simulink model "main"  (R2022b)
settings: Solver=FixedStepDiscrete  StartTime=0.0  StopTime=30  FixedStep=0.005  RelTol=1e-3
libraries: lib_button x1, simulink x1
settings Model: ExtModeTrigDuration=2  Creator=F64236C  LastModifiedBy=F64236C
settings OptimizationCC: EnhancedBackFolding=on  PassReuseOutputArgsAs=Individual arguments  ZeroExternalMemoryAtStartup=off  ZeroInternalMemoryAtStartup=off  MaxStackSize=64  OptimizeBlockOrder=speed  DifferentSizesBufferReuse=on  OptimizationCustomize=off  EfficientTunableParamExpr=on
settings DebuggingCC: ParameterTunabilityLossMsg=error
settings HardwareCC: ProdBitPerInt=16  ProdBitPerPointer=16  ProdBitPerSizeT=16  ProdBitPerPtrDiffT=16  ProdLargestAtomicFloat=None  ProdWordSize=8  ProdHWDeviceType=Atmel->AVR
settings SFSimCC: MATLABDynamicMemAlloc=off
settings RTWCC: Description=Embedded Coder  SystemTargetFile=ert.tlc  HardwareBoard=Arduino Uno  TLCOptions=-aInlineSetEventsForThisBaseRateFcn=TLC_FALSE -aSuppressMultiTaskScheduler=TLC_FALSE -aRateBasedStepFcn=1  TemplateMakefile=ert_default_tmf  Toolchain=Arduino AVR  BuildConfiguration=Faster Runs
settings CodeAppCC: ForceParamTrailComments=on  IgnoreCustomStorageClasses=off  OperatorAnnotations=on  SimulinkDataObjDesc=on  SFDataObjDesc=on  InsertBlockDesc=on
settings ERTTargetCC: SupportContinuousTime=on  SupportVariableSizeSignals=on  ExtModeTransport=3  ExtModeStaticAlloc=on  ExtModeAutomaticAllocSize=off  ExtModeStaticAllocSize=250  ExtModeMexFile=ext_xcp  ExtModeIntrfLevel=Level2 - Open

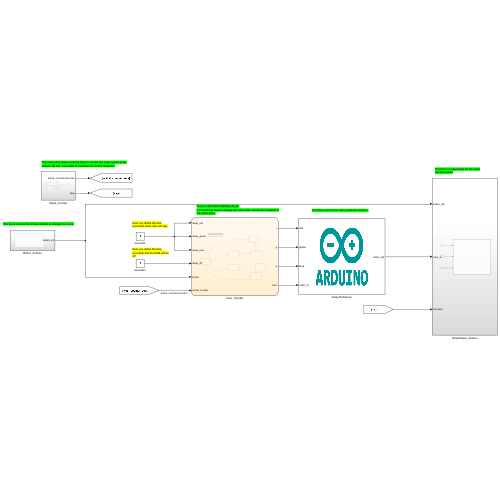
[thumbnail: Simulink's stored preview of the top-level diagram]
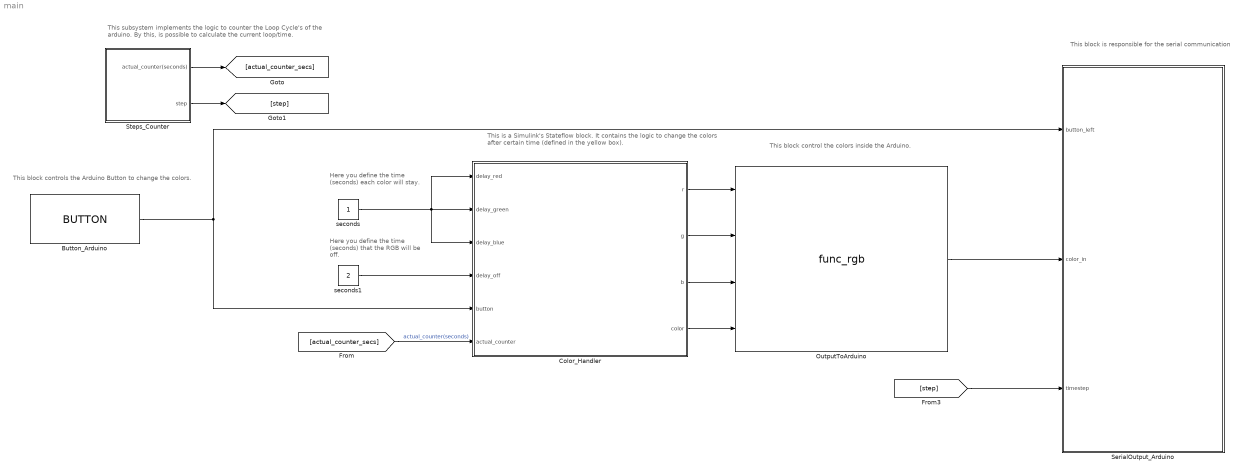
== system main ==
  note: Here you define the time (seconds) each color will stay.
  note: This is a Simulink's Stateflow block.
      | It contains the logic to change the colors after certain time (defined in the yellow box).
  note: Here you define the time (seconds) that the RGB will be off.
  note: This subsystem implements the logic to counter the Loop Cycle's of the arduino. By this, is possible to calculate the current loop/time.
  note: This block control the colors inside the Arduino.
  note: This block is responsible for the serial communication
  note: This block controls the Arduino Button to change the colors.
  Button_Arduino : lib_button/BUTTON  Priority=1  SystemSampleTime=-1  VariantActivationTime=update diagram  Latency=0  AutoFrameSizeCalculation=off
      link override S-Function Builder: FunctionName=func_button  SFunctionModules=func_button_wrapper.cpp
  Color_Handler : Stateflow chart  TreatAsAtomicUnit=on
  OutputToArduino : S-Function  FunctionName=func_rgb  SFunctionModules=func_rgb_wrapper.cpp  SFunctionDeploymentMode=off  EnableBusSupport=off  mask(S-Function Builder){}
      mask help: Simulink:masks:SFunctionBuilder_MD
      mask init:
      | val = [[.9  0.75 0.75 1 1 .9 .9 1]',[1 1 0.75 0.75 .9 .9 1 .9]'];try , sys = get_param(gcb,'SfunBuilderFcnName');if isempty(sys), sys = get_param(gcb,'FunctionName'); end,catch, sys = get_param(gcb,'FunctionName'); end
      settings: CopyFcn=set_param(gcbh,'LinkStatus','none')  OpenFcn=sfunctionwizard(gcbh)
      mask Display:
      | image('../imgs/arduino_logo.png');
      | 
      | %plot(val(:,1),val(:,2))
      | %disp(sys)
      | port_label('input',1,'red')
      | port_label('input',2,'green')
      | port_label('input',3,'blue')
      | port_label('input',4,'color_in')
      | port_label('output',1,'color_out')
  SerialOutput_Arduino : Subsystem  Priority=3
  Steps_Counter : Subsystem
  seconds : Constant  OutDataTypeStr=uint16
  seconds1 : Constant  Value=2  OutDataTypeStr=uint16
  wires:
  [actual_counter_secs] -> Color_Handler/6(actual_counter)  "actual_counter(seconds)"
  [step] -> SerialOutput_Arduino/3(timestep)
  seconds1/1 -> Color_Handler/4(delay_off)
  Steps_Counter/1(actual_counter(seconds)) -> [actual_counter_secs]
  Steps_Counter/2(step) -> [step]
  Button_Arduino/1 -> Color_Handler/5(button), SerialOutput_Arduino/1(button_left)
  seconds/1 -> Color_Handler/3(delay_blue), Color_Handler/1(delay_red), Color_Handler/2(delay_green)
  Color_Handler/1(r) -> OutputToArduino/1
  Color_Handler/2(g) -> OutputToArduino/2
  Color_Handler/3(b) -> OutputToArduino/3
  Color_Handler/4(color) -> OutputToArduino/4
  OutputToArduino/1 -> SerialOutput_Arduino/2(color_in)

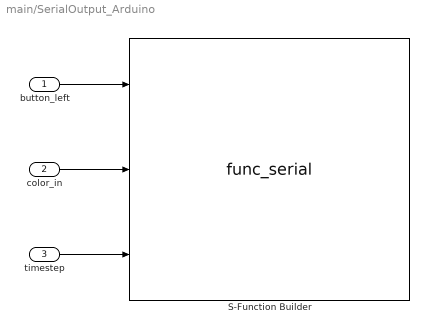
== system main/SerialOutput_Arduino ==
  button_left : Inport
  color_in : Inport  Port=2
  timestep : Inport  Port=3
  S-Function Builder : S-Function  FunctionName=func_serial  SFunctionModules=func_serial_wrapper.cpp  SFunctionDeploymentMode=off  EnableBusSupport=off  mask(S-Function Builder){}
      mask help: Simulink:masks:SFunctionBuilder_MD
      mask init: same as main/OutputToArduino
      settings: CopyFcn=set_param(gcbh,'LinkStatus','none')  OpenFcn=sfunctionwizard(gcbh)
      mask Display:
      | plot(val(:,1),val(:,2))
      | disp(sys)
      | port_label('input',1,'button_left')
      | port_label('input',2,'color_in')
      | port_label('input',3,'timestep')
  wires:
  timestep/1 -> S-Function Builder/3
  button_left/1 -> S-Function Builder/1
  color_in/1 -> S-Function Builder/2

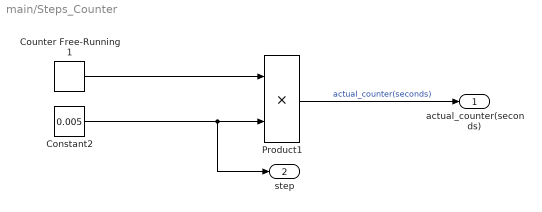
== system main/Steps_Counter ==
  Constant2 : Constant  Value=0.005
  Counter Free-Running1 : simulink/Sources/Counter Free-Running  NumBits=32  tsamp=-1
  Product1 : Product  OutDataTypeStr=double
  actual_counter(seconds) : Outport
  step : Outport  Port=2
  wires:
  Constant2/1 -> step/1, Product1/2
  Counter Free-Running1/1 -> Product1/1
  Product1/1 -> actual_counter(seconds)/1  "actual_counter(seconds)"

== stateflow chart main/Color_Handler ==
  state y = delay(start_counter, duration) [function]
    (default) -> (junction 81)
    (junction 81) -> (junction 82) [order 1] : [(actual_counter - start_counter) >= duration]
    (junction 82) -> (junction 71) : {y=true}
    (junction 81) -> (junction 73) [order 2]
    (junction 73) -> (junction 71) : {y=false}
  state blue_fraco
    en:
    r = 0;
    g = 0;
    b = 128;
    color = 3;
    counter_blue = actual_counter;
  state red_fraco
    en:
    r = 255;
    g = 180;
    b = 180;
    color = 1;
    counter_red = actual_counter;
  state green_fraco
    en:
    r = 0;
    g = 128;
    b = 0;
    color = 2;
    counter_green = actual_counter;
  state off
    en:
    r = 0;
    g = 0;
    b = 0;
    color = 0;
    counter_off = actual_counter;
  state green_forte
    en:
    r = 0;
    g = 255;
    b = 0;
    color = 2;
    counter_green = actual_counter;
  state red_forte
    en:
    r = 255;
    g = 0;
    b = 0;
    color = 1;
    counter_red = actual_counter;
  state blue_forte
    en:
    r = 0;
    g = 0;
    b = 255;
    color = 3;
    counter_blue = actual_counter;
  blue_fraco -> off : [delay(counter_blue,delay_blue)]
  green_fraco -> blue_fraco : [delay(counter_green,delay_green)]
  red_fraco -> green_fraco : [delay(counter_red,delay_red) ]
  off -> red_fraco [order 2] : [delay(counter_off,delay_off) && ~button]
  (default) -> off
  blue_forte -> off : [delay(counter_blue,delay_blue)]
  off -> red_forte [order 1] : [delay(counter_off,delay_off) && button]
  red_forte -> green_forte : [delay(counter_red,delay_red)]
  green_forte -> blue_forte : [delay(counter_green,delay_green) ]
  data: start_counter function_input; duration function_input; y function_output; delay_red input uint16; delay_green input uint16; r output uint16; g output uint16; delay_blue input uint16; delay_off input uint16; b output uint16; color output uint16; button input boolean; actual_counter input double; counter_off local double; counter_blue local double; counter_green local double; counter_red local double
